simulink library "common_lib"  (R2023a)
settings: Solver=ode45  StartTime=0.0  StopTime=10.0  RelTol=1e-3
undefined symbols (not defined in the file): ACCEL_PRE_MULT, APDT_SrvcMgr_IRVHVDCSubFcnReq, C_C1GearNumbers, C_C1GearRatios, C_Calibration, C_DitherWaveform, C_GearOffset, C_GearRatioIn, C_GearRatioInverseOut, C_GearRatioOut, CLUTCH_INNER_LOOP_UPDATE_RATE, CONSTANT, DEGRADED_MODE_SIZE, Dem_EventStatusType, DiscIntNeverNeededParam, F_FAULT_ENUM, F_NOFAULT, F_OUTOFRANGE, F_RATELIMIT, FALSE, FMI14_SPECIAL_INSTRUCTIONS, FMI20_DATA_DRIFTED_HIGH, FMI21_DATA_DRIFTED_LOW, FMI29_RESERVED_FOR_SAE_ASSIGNMENT, FMI30_RESERVED_FOR_SAE_ASSIGNMENT, FMI31_CONDITION_EXISTS, FMI32_NO_FAULT, IC, k_accel, k_mean, MAX_UINT32, MEAN_PRE_MULT, NTriggers, QLTY_SIGNAL_FAILED, QLTY_SIGNAL_FULLY_FUNCTION, QLTY_SIGNAL_SUBSTITUTED_BY_1ST_CHOICE, QLTY_SIGNAL_SUBSTITUTED_BY_2ND_CHOICE, QLTY_SIGNAL_SUBSTITUTED_BY_3RD_CHOICE, QLTY_SIGNAL_SUBSTITUTED_BY_4TH_CHOICE, SAMPLE_TIME_100us, SAMPLETIME_10ms_Int, SATURATION_U16, simin, T_TestPoint, TF_FALSE, TF_TRUE, TimeStep, TRUE, WORKSPACE_UPDATE_RATE, ZERO, Zero
libraries: $bdroot x123, simulink x28, simulink_extras x4, MBD_EPS_Local_Blockset x4
(part 3 of 10)

== system common_lib/Misc ==
  note: Miscellaneous Computations
  ArcSine : Subsystem  mask(CL Trigonometric Function ArcSine){}
      mask help:
      | Simple trigonometric arcsine function.  The sine is the input and the angle is the output.
      |
      | This block is single precision.  The calculation used to determine arcsine is dervied from a Taylor Series approximation.  Note there are limitations with this approximation such as round off error.
      |
      | NgEK, Inc.
      mask Help: web(which(['common_lib51.html']))
      mask Display:
      | patch([0.30 0.30 0.70 0.70], [0.25 0.75 0.75 0.25], [255/255 127/255 255/255])
      | plot(linspace(-1,1,20)/6+0.5,(asin(linspace(-1,1,20)))/6.28+0.5)
  ClampAboveZero : Subsystem  mask(CL Clamp Above Zero){Tol=[]}
      mask prompts: Tol "Tolerance"
      mask help:
      | Clamps input above zero according to a calibratible tolerance.
      |
      | X(1) = input
      |
      | Y(1) = output
      | NgEK, Inc.
      settings: AttributesFormatString=tol=%<Tol>
      mask Help: web(which(['common_lib21.html']))
      mask Display:
      | patch([0.3 0.3 0.7 0.7], [0.35 0.65 0.65 0.35], [255/255 127/255 255/255])
      | 
      | plot([0 1],[0.5 0.5], [0.5 0.5],[0 1], [0 0.5 1], [0.55 0.55 1])
  ClampAroundZero : Subsystem  mask(CL Clamp Around Zero){Tol=[]}
      mask prompts: Tol "Tolerance"
      mask help:
      | Clamps input around zero according to a calibratible tolerance.
      |
      | X(1) = input
      |
      | Y(1) = output
      | NgEK, Inc
      mask init:
      | switch class(Tol)
      |   case ('double')
      |       One      = double(1.0);
      |        Zero     = double(0.0);
      |        MinusOne = double(-1.0);
      |  case ('single')
      |         One      = single(1.0);
      |        Zero     = single(0.0);
      |          MinusOne = single(-1.0);
      |  case ('int8')
      |         One      = int8(1.0);
      |          Zero     = int8(0.0);
      |          MinusOne = int8(-1.0);
      |     case ('int16')
      |        One      = int16(1.0);
      |         Zero     = int16(0.0);
      |         MinusOne = int16(-1.0);
      |   case ('int32')
      |         One      = int32(1.0);
      |         Zero     = int32(0.0);
      |         MinusOne = int32(-1.0);
      | end;
      settings: AttributesFormatString=tol=%<Tol>
      mask Help: web(which(['common_lib22.html']))
      mask Display:
      | patch([0.3 0.3 0.7 0.7], [0.35 0.65 0.65 0.35], [255/255 127/255 255/255])
      | 
      | plot([0 1],[0.5 0.5], [0.5 0.5],[0 1], [0 0.3 0.5 0.5 0.7 1], [0 0.3 0.3 0.7 0.7 1])
  Cosine : Subsystem  mask(CL Trigonometric Function Cosine){}
      mask help:
      | Simple trigonometric cosine function.  The angle is the input and the cosine angle is the output.
      |
      | This block is single precision.  The calculation used to determine cosine is dervied from a Taylor Series approximation.  Note there are limitations with this approximation such as round off error.
      |
      | NgEK, Inc.
      mask Help: web(which(['common_lib52.html']))
      mask Display:
      | patch([0.30 0.30 0.70 0.70], [0.25 0.75 0.75 0.25], [255/255 127/255 255/255])
      | plot(linspace(0,6.28,20)/16+0.3,(1+cos(linspace(0,6.28,20)))/4+0.25)
  Count Edges : Subsystem  mask(CL Count Edges){}
      mask help:
      | Generic counter
      |
      | Counts the number of edges from FALSE to TRUE.  Includes reset input to set the count back to zero.
      mask Help: web(which(['common_lib54.html']))
      mask Display:
      | patch([0.30 0.30 0.70 0.70], [0.25 0.75 0.75 0.25], [255/255 127/255 255/255])
      | disp('Count Edges')
  Count to X : Subsystem  mask(CL Count To X){X=[], edge=FALSE to TRUE}
      mask prompts: X "Divide by count"; edge "Count edge"
      mask help:
      | Generic count to X
      | Outputs a TRUE after X edges.
      |
      | Edge polarity and X are set by mask.
      | NgEK, Inc.
      mask init:
      | h_input      = [gcb '/Input'];
      | h_dinput    = [gcb '/DelayedInput'];
      | 
      | switch get_param(gcb,'edge')
      |    case 'FALSE to TRUE'
      |       set_param(h_input,  'Operator','AND');
      |         set_param(h_dinput, 'Operator','NAND');
      |  otherwise
      |      set_param(h_input,  'Operator','NAND');
      |         set_param(h_dinput, 'Operator','AND');
      | end
      mask Help: web(which(['common_lib26.html']))
      mask TypeOptions edge: FALSE to TRUE | TRUE to FALSE
      mask Display:
      | patch([0.1 0.1 0.9 0.9], [0.2 0.8 0.8 0.2], [255/255 127/255 255/255])
      | disp([...
      |        'Count to ' get_param(gcb,'X') '\n'...
      |        get_param(gcb,'edge')...
      |   ])
      | port_label('input',1,'in');
      | port_label('input',2,'reset?');
      | port_label('output',1,'out');
  Counter : Subsystem  mask(CL Counter){IC=[]}
      mask prompts: IC "Initial condition"
      mask help:
      | Generic counter block.
      | Counts up by up_val when count_up? is true
      | Counts down by down_val when count_down? is true.
      | Block can be used as a timer if increment value is set to the frame rate.
      |
      | X(1) = increment value
      | X(2) = count up flag
      | X(3) = decrement value
      | X(4) = count down flag
      | X(5) = max counter value
      | X(6) = min counter value
      | X(7) = reset
      |
      | Y(1) = output
      |
      | Initial condition is entered via mask.
      | NgEK, Inc.
      mask init:
      | switch class(IC)
      |    case ('double')
      |         Zero     = double(0.0);
      |   case ('single')
      |        Zero     = single(0.0);
      |   case ('int8')
      |       Zero     = int8(0.0);
      |     case ('uint16')
      |        Zero     = uint16(0.0);
      |  case ('uint32')
      |         Zero     = uint32(0.0);
      |     case ('int16')
      |         Zero     = int16(0.0);
      |    case ('int32')
      |         Zero     = int32(0.0);
      | end;
      mask Help: web(which(['common_lib23.html']))
      mask Display:
      | patch([0.4 0.4 0.6 0.6], [0.4 0.6 0.6 0.4], [255/255 127/255 255/255])
      | disp('Counter')
      | port_label('input', 1, 'up_val')
      | port_label('input', 2, 'count_up?')
      | port_label('input', 3, 'down_val')
      | port_label('input', 4, 'count_down?')
      | port_label('input', 5, 'max_count')
      | port_label('input', 6, 'min_count')
      | port_label('input', 7, 'reset?')
      | port_label('output', 1, 'output')
  Divide by X : Subsystem  mask(CL Divide By X){X=[]}
      mask prompts: X "Divide by count"
      mask help:
      | Generic divide by X
      | Outputs a true every X iterations.
      |
      | trigger? input forces output true
      |
      | Divide by X  is entered via mask.
      | NgEK, Inc.
      mask Help: web(which(['common_lib25.html']))
      mask Display:
      | patch([0.3 0.3 0.7 0.7], [0.4 0.6 0.6 0.4], [255/255 127/255 255/255])
      | disp(['Divide by ' num2str(X)])
      | port_label('input', 1, 'trigger?')
      | port_label('output', 1, 'output')
  EatonLogo : Subsystem
      mask Display: image(imread('EatonLogo.jpg'));
  EdgeTriggered Pulse : Subsystem  RTWFcnName=ETP  mask(CL Edge Triggered Pulse){Edge=TRUE to FALSE, Width=[], Pulse=TRUE, TimeStep=[], Init=0}
      mask prompts: Edge "Edge Detection"; Width "Pulse Width (seconds)"; Pulse "Pulse Value (boolean)"; TimeStep "Time Step"; Init "N/A"
      mask help:
      | Upon detection of an edge on the input (TRUE to FALSE or FALSE to TRUE)
      | output a pulse (TRUE or FALSE).
      |
      | Edge detect, pulse value, pulse width and update rate (the last two are SINGLE type) are entered via the mask.
      | NgEK, Inc.
      mask init:
      | set_param([gcb '/ETP'],'Edge',get_param(gcb,'Edge'));
      | set_param([gcb '/ETP'],'Pulse',get_param(gcb,'Pulse'));
      | set_param([gcb '/ETP'],'TimeStep',get_param(gcb,'TimeStep'));
      settings: RTWFcnNameOpts=User specified  RTWFileNameOpts=Use function name
      mask Help: web(which(['common_lib28.html']))
      mask TypeOptions Edge: FALSE to TRUE | TRUE to FALSE
      mask TypeOptions Pulse: TRUE | FALSE
      mask Display:
      | patch([0.02 0.02 0.98 0.98], [0.1 0.9 0.9 0.1], [255/255 127/255 255/255]);
      | disp([...
      |       'Edge= ' get_param(gcb,'edge') '\n'...
      |       'Width= ' get_param(gcb,'width') '\n'...
      |       'Pulse Value= ' get_param(gcb,'pulse')...
      |  ]);
  EdgeTriggered Pulse w time : Subsystem  RTWFcnName=ETPWT  mask(CL Edge Triggered Pulse w Time){Edge=TRUE to FALSE, Pulse=FALSE, TimeStep=[], Init=0}
      mask prompts: Edge "Edge Detection"; Pulse "Pulse Value (boolean)"; TimeStep "Time Step"; Init "N/A"
      mask help:
      | Upon detection of an edge on the input (TRUE to FALSE or FALSE to TRUE)
      | output a pulse (TRUE or FALSE).
      |
      | Edge detect, pulse value, pulse width and update rate (the last two are SINGLE type)
      | are entered via the mask.
      | NgEK, Inc.
      mask init:
      | switch get_param(gcb,'Edge')
      |     case 'FALSE to TRUE'
      |        TRIGGER=false;
      |    otherwise
      |        TRIGGER=true;
      | end
      | 
      | switch get_param(gcb,'Pulse')
      |    case 'FALSE'
      |       OUTPUT = false;
      |    otherwise
      |       OUTPUT = true;
      | end
      | Ts = single(TimeStep);
      | Ts_half = Ts/single(2.0);
      settings: RTWSystemCode=Inline  RTWFcnNameOpts=User specified  RTWFileNameOpts=Use function name
      mask Help: web(which(['common_lib29.html']))
      mask TypeOptions Edge: FALSE to TRUE | TRUE to FALSE
      mask TypeOptions Pulse: TRUE | FALSE
      mask Display:
      | patch([0.02 0.02 0.98 0.98], [0.1 0.9 0.9 0.1], [255/255 127/255 255/255]);
      | disp([...
      |       'Edge= ' get_param(gcb,'edge') '\n'...
      |       'Pulse Value= ' get_param(gcb,'pulse')...
      |     ]);
  GreenLeaf_Globe : Subsystem
      mask Display: image(imread('greenleaf_globe.png'));
  Hold : Subsystem  TreatAsAtomicUnit=on
      settings: RTWSystemCode=Inline
      mask Display:
      | patch([0.25 0.25 0.75 0.75], [0.05 0.3 0.3 0.05], [255/255 127/255 255/255])
      | disp('\n\nHold');
  Latch : Subsystem  mask(CL Latch){IC=[]}
      mask prompts: IC "Initial Condition"
      mask help:
      | Input is latched until reset is true
      |
      | X(1) = input
      | X(2) = reset
      |
      | Y(1) = output
      |
      | Initial condition is entered via mask.
      | NgEK, Inc.
      mask Help: web(which(['common_lib24.html']))
      mask Display:
      | patch([0.35 0.35 0.65 0.65], [0.3 0.65 0.65 0.3], [255/255 127/255 255/255])
      | disp('Latch')
      | port_label('input', 1, 'input')
      | port_label('input', 2, 'reset?')
      | port_label('output', 1, 'output')
  ModelVersion : Subsystem  mask{Parameter1=0}
      mask init:
      | % Use the simulink model verison
      | mdlName = get_param(bdroot,'name'); 
      | mdlVersionStr = get_param(bdroot,'Modelversion');
      | mdlVersion = single(str2num(mdlVersionStr));
      | mdlVersionSignal =[strrep(mdlName,'SWC_','') '_SwcVer'];
      | 
      | %Set the signal name to match the SwC
      | p = get_param([gcb '/mdlVersionBlock'],'PortHandles');
      | l = get_param(p.Outport,'Line');
      | set_param(l,'Name',mdlVersionSignal);
      | set_param(p.Outport,'MustResolveToSignalObject','on');
      | 
      | %Open the data dictionary
      | try
      |     myDictionaryObj = ...
      |     Simulink.data.dictionary.open([mdlName '.sldd']);
      |     dDataSectObj = getSection(myDictionaryObj,'Design Data');
      | 
      |     %Check if the signal object is present
      |     %foundEntries = find(dDataSectObj,'Name',mdlVersionSignal,'-class','Simulink.Signal');
      | 
      |     if ~exist(dDataSectObj,mdlVersionSignal)
      |         entryDiction = addEntry(dDataSectObj,mdlVersionSignal,Simulink.Signal);
      |         entrySub = Simulink.Signal;
      |         entrySub.DataType = 'single';
      |         entrySub.Min = 0;
      |         entrySub.CoderInfo.StorageClass = 'ExportedGlobal'
      |         setValue(entryDiction,entrySub);
      |         saveChanges(myDictionaryObj);
      |     end        
      |     close(myDictionaryObj); 
      |     
      | catch
      |     
      | end
      mask DialogControl DescTextVar Prompt: This model adds correct signal object to display the correct model version
      mask Display: disp('Model Version')
  NonZero : Subsystem  mask(CL Non Zero){Tol=0}
      mask prompts: Tol "Tolerance"
      mask help:
      | Determines whether the input is within tolerance of zero.
      |
      | Outputs a Boolean
      | TRUE means the value is non-zero
      | FALSE means the value is within tolerance of zero
      mask Display:
      | patch([0.1 0.3 0.2 0.2], [0.4 0.6 0.6 0.4], [255/255 127/255 255/255])
      | 
      | disp([...
      |       'Non-Zero\n'...
      |       'tol= ' get_param(gcb,'Tol')...
      |  ]);
  Sine : Subsystem  mask(CL Trigonometric Function Sine){}
      mask help:
      | Simple trigonometric sine function.  The angle is the input and the sine angle is the output.
      |
      | This block is single precision.  The calculation used to determine sine is dervied from a Taylor Series approximation.  Note there are limitations with this approximation such as round off error.
      |
      | NgEK, Inc.
      mask Help: web(which(['common_lib51.html']))
      mask Display:
      | patch([0.30 0.30 0.70 0.70], [0.25 0.75 0.75 0.25], [255/255 127/255 255/255])
      | plot(linspace(0,6.28,20)/16+0.3,(1+sin(linspace(0,6.28,20)))/4+0.25)
  Tangent : Subsystem  mask(CL Trigonometric Function Sine){}
      mask help:
      | Simple trigonometric tangent function.  The angle is the input and the tan angle is the output.
      |
      | This block is single precision.  The calculation used to determine tangent is dervied from a Taylor Series approximation.  Note there are limitations with this approximation such as round off error.
      |
      | NgEK, Inc.
      mask Help: web(which(['common_lib53.html']))
      mask Display:
      | patch([0.30 0.30 0.70 0.70], [0.25 0.75 0.75 0.25], [255/255 127/255 255/255])
      | plot(linspace(0,6.28,20)/16+0.3,(1+tan(linspace(0,6.28,20)))/10+0.25)
  Timeout Detection : Subsystem  RTWFcnName=TIMEOUT  mask(CL Timeout){Timeout=[], TimeStep=[]}
      mask prompts: Timeout "Timeout  (seconds)"; TimeStep "Time Step"
      mask help:
      | Timeout detection monitors the input
      | and signals a TRUE if the input is unchanging
      | for longer than the timeout interval.
      |
      | Update Rate and Timeout are entered via the mask.
      | NgEK, Inc.
      mask init:
      | % switch class(Timeout)
      | %   case ('double')
      | %        Tol      = double(TimeStep)/2.0;
      | %       Zero     = double(0.0);
      | %   case ('single')
      | %         Tol      = single(double(TimeStep)/2.0);
      | %         Zero     = single(0.0);
      | %    case ('int8')
      | %       Tol      = int8(double(TimeStep)/2.0);
      | %          Zero     = int8(0.0);
      | %     case ('int16')
      | %         Tol      = int16(double(TimeStep)/2.0);        
      | %       Zero     = int16(0.0);
      | %    case ('int32')
      | %          Tol      = int32(double(TimeStep)/2.0);       
      | %        Zero     = int32(0.0);
      | % end;
      | 
      | Ts = single(TimeStep);
      | Tol = Ts/single(2.0);
      | Zero = single(0.0);
      settings: RTWFcnNameOpts=User specified  RTWFileNameOpts=Use function name
      mask Help: web(which(['common_lib27.html']))
      mask Display:
      | patch([0.05 0.05 0.95 0.95], [0.15 0.85 0.85 0.15], [255/255 127/255 255/255]);
      | disp(['Timeout = \n' get_param(gcb,'Timeout')]);
  Timeout with time : Subsystem  RTWFcnName=TIMEOUT  mask(CL Timeout){TimeStep=[]}
      mask prompts: TimeStep "Time Step"
      mask help:
      | Timeout detection monitors the input
      | and signals a TRUE if the input is unchanging
      | for longer than the timeout interval.
      |
      | Update Rate and Timeout are entered via the mask.
      | NgEK, Inc.
      mask init: same as common_lib/Misc/Timeout Detection
      settings: RTWFcnNameOpts=User specified  RTWFileNameOpts=Use function name
      mask Help: web(which(['common_lib27.html']))
      mask Display:
      | patch([0.05 0.05 0.95 0.95], [0.15 0.85 0.85 0.15], [255/255 127/255 255/255]);
      | disp(['Timeout = \n Input Port 2' ]);
  Timeout with time Integer : Subsystem  RTWFcnName=TIMEOUT  mask(CL Timeout){TimeStep=[]}
      mask prompts: TimeStep "Time Step"
      mask help:
      | Timeout detection monitors the input
      | and signals a TRUE if the input is unchanging
      | for longer than the timeout interval.
      |
      | Update Rate and Timeout are entered via the mask.
      | NgEK, Inc.
      mask init:
      | % switch class(Timeout)
      | %   case ('double')
      | %        Tol      = double(TimeStep)/2.0;
      | %       Zero     = double(0.0);
      | %   case ('single')
      | %         Tol      = single(double(TimeStep)/2.0);
      | %         Zero     = single(0.0);
      | %    case ('int8')
      | %       Tol      = int8(double(TimeStep)/2.0);
      | %          Zero     = int8(0.0);
      | %     case ('int16')
      | %         Tol      = int16(double(TimeStep)/2.0);        
      | %       Zero     = int16(0.0);
      | %    case ('int32')
      | %          Tol      = int32(double(TimeStep)/2.0);       
      | %        Zero     = int32(0.0);
      | % end;
      | 
      | Ts = uint16(TimeStep);
      | Tol = uint16(Ts/uint16(2));
      | Zero = uint16(0);
      settings: RTWFcnNameOpts=User specified  RTWFileNameOpts=Use function name
      mask Help: web(which(['common_lib27.html']))
      mask Display:
      | patch([0.05 0.05 0.95 0.95], [0.15 0.85 0.85 0.15], [255/255 127/255 255/255]);
      | disp(['Int_Timeout = \n Input Port 2' ]);
  Value Latch1 : Subsystem  mask(CL Latch){IC=[], HoldTime=0, TimeStep=0}
      mask prompts: IC "Initial Condition"; HoldTime "Hold Time"; TimeStep "Time Step"
      mask help:
      | Input is latched until reset is true
      |
      | X(1) = input
      | X(2) = reset
      |
      | Y(1) = output
      |
      | Initial condition is entered via mask.
      | NgEK, Inc.
      mask Help: web(which(['common_lib24.html']))
      mask Display:
      | patch([0.35 0.35 0.65 0.65], [0.3 0.65 0.65 0.3], [255/255 127/255 255/255])
      | disp('Latch')
      | port_label('input', 1, 'input')
      | port_label('output', 1, 'output')

== system common_lib/OS ==
  note: These components are atomic elements used by the
      | schedule_morph script to build scheduler blocks
  note: OS Components
  Scheduler : Subsystem  mask(CL Scheduler){Number=5, DType=Fcn_Call, Style=Trigger all tasks each frame, State=off}
      mask prompts: Number "Number of Tasks to Trigger"; DType "Type of Trigger"; Style "Schedule Style"; State "Display Scheduler State"
      mask help:
      | Simulink-based task scheduler capable of generating  boolean or fcn_call triggers.  Tasks may be staggered so that one is executed each frame in a round-robin fashion or all tasks may be triggered in sequence in a single frame.
      |
      | Boolean output for all tasks triggering in a frame is not implemented yet.
      |
      | NgEK, Inc.
      mask init:
      | NTriggers=int8(max([Number 1]));
      | TRUE = boolean(1);
      | FALSE = boolean(0);
      | schedule_morph;
      settings: RTWSystemCode=Nonreusable function  RTWFcnNameOpts=Use subsystem name  RTWFileNameOpts=Use subsystem name
      mask Help: web(which(['common_lib30.html']))
      mask TypeOptions DType: Boolean | Fcn_Call
      mask TypeOptions Style: Trigger one task per frame | Trigger all tasks each frame
      mask Display:
      | patch([0.3 0.3 0.7 0.7], [0.35 0.65 0.65 0.35], [255/255 127/255 255/255])
      | disp('Scheduler');
      | 
      | port_label('output',1,'Task 1');
      | port_label('output',2,'Task 2');
      | port_label('output',3,'Task 3');
      | port_label('output',4,'Task 4');
      | port_label('output',5,'Task 5');
  Scheduler with Init : Subsystem  mask(CL Scheduler with Init){Number=2}
      mask prompts: Number "Number of Tasks to Trigger"
      mask help:
      | Simulink-based task scheduler capable of generating  fcn_call triggers.  Tasks are triggered in sequence in a single frame.  The task wired to the "Init" port is only executed in the first frame.
      |
      | NgEK, Inc.
      mask init:
      | NTriggers=int8(max([Number 1]));
      | TRUE = boolean(1);
      | FALSE = boolean(0);
      | schedule_morph2;
      settings: RTWSystemCode=Nonreusable function  RTWFcnNameOpts=Use subsystem name  RTWFileNameOpts=Use subsystem name
      mask Help: web(which(['common_lib55.html']))
      mask Display:
      | patch([0.3 0.3 0.7 0.7], [0.35 0.65 0.65 0.35], [255/255 127/255 255/255])
      | disp('Scheduler\nwith Init');
      | 
      | port_label('output',1,'Init');
      | port_label('output',2,'Task 1');
      | port_label('output',3,'Task 2');
  fcn_call generator : Subsystem  TreatAsAtomicUnit=on
  schedule counter : Subsystem
  sequence generator : Subsystem  TreatAsAtomicUnit=on

== system common_lib/SCond ==
  note: Signal Conditioning
  Gain and Offset (in) : Subsystem  mask(CL Gain And Offset (in)){DataType=Single}
      mask prompts: DataType "Output Data Type"
      mask help:
      | Gain/Offset with data type coercion
      |
      | NgEK, Inc.
      mask init:
      | h=gcb;
      | 
      | set_param([h '/InputConversion'], 'DataType','single');
      | set_param([h '/InputConversion1'], 'DataType','single');
      | set_param([h '/InputConversion2'], 'DataType','single');
      | 
      | switch DataType
      |   case (1)
      |       set_param([h '/OutputConversion'], 'DataType','int8');
      |  case (2)
      |       set_param([h '/OutputConversion'], 'DataType','uint8');
      |    case (3)
      |       set_param([h '/OutputConversion'], 'DataType','int16');
      |  case (4)
      |      set_param([h '/OutputConversion'], 'DataType','uint16');
      |   case (5)
      |         set_param([h '/OutputConversion'], 'DataType','single');
      |    case (6)
      |         set_param([h '/InputConversion'], 'DataType','double');
      |         set_param([h '/InputConversion1'], 'DataType','double');
      |         set_param([h '/InputConversion2'], 'DataType','double');
      |      set_param([h '/OutputConversion'], 'DataType','double');    
      |    otherwise
      |      set_param([h '/OutputConversion'], 'DataType','single');
      | end
      mask Help: web(which(['common_lib32.html']))
      mask TypeOptions DataType: Int8 | UInt8 | Int16 | UInt16 | Single | Double
      mask Display:
      | patch([0.35 0.35 0.65 0.65], [0.35 0.65 0.65 0.35], [255/255 127/255 255/255]);
      | disp(['mx-b']);
  Gain and Offset (out) : Subsystem  mask(CL Gain And Offset (out)){DataType=Single}
      mask prompts: DataType "Output Data Type"
      mask help:
      | Gain/Offset with data type coercion
      |
      | NgEK, Inc.
      mask init: same as common_lib/SCond/Gain and Offset (in)
      mask Help: web(which(['common_lib33.html']))
      mask TypeOptions DataType: Int8 | UInt8 | Int16 | UInt16 | Single | Double
      mask Display:
      | patch([0.35 0.35 0.65 0.65], [0.35 0.65 0.65 0.35], [255/255 127/255 255/255]);
      | disp(['(x+b)/m']);
  Membership Function : Subsystem  mask(CL Membership Function){Low=single(10), Peak=single(50), High=single(90), DType=Upper Trapezoid}
      mask prompts: Low "Lower Value"; Peak "Peak Value"; High "Upper Value"; DType "Membership Type"
      mask help:
      | Triangular membership function calculation with an output of 1 at the "Peak" value and dropping off to 0 towards the "Low" and "High" values.  End "trapezoid" membership functions may be specified with the membership "type" pulldown menu.
      |
      | X(1) = Independent Variable
      |
      | Y(1) = Membership Function (0:1)
      |
      | NgEK, Inc.
      mask init:
      | if Peak<Low | Peak>High, disp(['WARNING: Breakpoints Non-Monotonic in <' gcb '>!']), end
      | 
      | switch class(Peak)
      |   case ('double')
      |        Zero      = double( 0.0);
      |          One       = double( 1.0);
      |         if (DType==1)
      |             SlopeLow  = 0.0;
      |           SlopeHigh = 1.0/(Peak-High);
      |         elseif (DType==2)
      |             SlopeLow  = 1.0/(Peak-Low);
      |            SlopeHigh = 1.0/(Peak-High);
      |       else
      |          SlopeLow  = 1.0/(Peak-Low);
      |           SlopeHigh = 0.0;
      |        end;
      |      
      |     case ('single')
      |        Zero      = single( 0.0);
      |          One       = single( 1.0);
      |        if (DType==1)
      |            SlopeLow  = single(0.0);
      |           SlopeHigh = single(1.0/(double(Peak)-double(High)));
      |          elseif (DType==2)
      |            SlopeLow  = single(1.0/(double(Peak)-double(Low)));
      |            SlopeHigh = single(1.0/(double(Peak)-double(High)));
      |       else
      |          SlopeLow  = single(1.0/(double(Peak)-double(Low)));
      |           SlopeHigh = single(0.0);
      |         end;
      | end;
      | 
      | if     (abs(double(SlopeLow))<abs(double(SlopeHigh)))
      |   XPltAxis = [ 0 0.2 0.7 0.8 1.0 ];
      | elseif (abs(double(SlopeHigh))<abs(double(SlopeLow)))
      |  XPltAxis = [ 0 0.2 0.3 0.8 1.0 ];
      | else
      |  XPltAxis = [ 0 0.2 0.5 0.8 1.0 ];
      | end;
      | 
      | if     (DType==1)
      |        YPltAxis = [ 1 1 0 0 0 ];
      | elseif (DType==2)
      |        YPltAxis = [ 0 0 1 0 0 ];
      | else
      |        YPltAxis = [ 0 0 0 1 1 ];
      | end;
      mask Help: web(which(['common_lib36.html']))
      mask TypeOptions DType: Lower Trapezoid | Central Triangle | Upper Trapezoid
      mask Display:
      | patch([.2 .2 .8 .8],[.2 .85 .85 .2],[255/255 127/255 255/255])
      | plot(XPltAxis, YPltAxis);
      | disp(['Low=',num2str(double(Low)),sprintf('\n'),'Peak=',num2str(double(Peak)),sprintf('\n'),'High=',num2str(double(High))])
  Test Override Gain and Offset (in) : Subsystem  mask(CL Gain And Offset (in)){DataType=Single}
      mask prompts: DataType "Output Data Type"
      mask help: Gain/Offset with enabled Gain and Offset option and with Output data type conversion
      mask init: same as common_lib/SCond/Gain and Offset (in)
      mask TypeOptions DataType: Int8 | UInt8 | Int16 | UInt16 | Single | Double
      mask Display:
      | patch([0.3 0.3 0.7 0.7], [0.35 0.65 0.65 0.35], [255/255 127/255 255/255])
      | disp(['Y=mX+b\nTest Override'])
  ramp to zero : Subsystem  mask(CL Ramp to Zero){DataType=Single}
      mask prompts: DataType "Data Type"
      mask help:
      | Ramp input signal to zero
      |
      | X(1) = Speed
      | X(2) = Limit
      |
      | Y(1) = Factor
      |
      | NgEK, Inc.
      mask init:
      | switch DataType
      |     case (1)
      |        One      = single( 1.0);
      |          MinusOne = single(-1.0);
      |         Zero     = single( 0.0);
      |     case (2)
      |         One      = double( 1.0);
      |          MinusOne = double(-1.0);
      |       Zero     = double( 0.0);
      | end;
      mask Help: web(which(['common_lib34.html']))
      mask TypeOptions DataType: Single | Double
      mask Display:
      | patch([0.3 0.3 0.7 0.7], [0.3 0.7 0.7 0.3], [255/255 127/255 255/255]);
      | disp('ramp to\nzero')

== system common_lib/Signal Conditioning ==
  note: Signal Conditioning
  2nd Order Butterworth Filter : Subsystem  mask{IC=0, TSAMP=0}
      mask prompts: IC "Initial Condition"; TSAMP "Sample Time"
      mask Display:
      | patch([0.35 0.35 0.65 0.65], [0.3 0.7 0.7 0.3], [255/255 127/255 255/255])
      | disp('2nd Order\nButterworth')
      | port_label('input',1,'input')
      | port_label('input',2,'cutoff_freq')
      | port_label('input',3,'reset')
      | port_label('output',1,'output')
  AnalogChecking : Subsystem  TreatAsAtomicUnit=on  mask{TimeStep=[]}
      mask prompts: TimeStep "Time Step"
  DitherSaturation : Subsystem  Description=|
      | This block generates dither using the table given for DitherWaveform at the frequency and amplitude given by the freq_hz and amplitude inputs.  All inputs should be 'single' datatype.  The table should be 'single' data type also.  The block runs at the sample time of the 'in' input.  It generates the correct frequency dither regardless of sample time.
      |                                                                                                                                                                                                                                                                                                                                                                  
      | Since it may not be possible to generate the exact frequency specified in the 'freq_hz' input, the block puts out the actual frequency in the 'realized_frequency' output.
  DitherSaturation1 : Subsystem  Description=|
      | This block generates dither using the table given for DitherWaveform at the frequency and amplitude given by the freq_hz and amplitude inputs.  All inputs should be 'single' datatype.  The table should be 'single' data type also.  The block runs at the sample time of the 'in' input.  It generates the correct frequency dither regardless of sample time.
      |                                                                                                                                                                                                                                                                                                                                                                  
      | Since it may not be possible to generate the exact frequency specified in the 'freq_hz' input, the block puts out the actual frequency in the 'realized_frequency' output.
  HydValveDither : Subsystem  Description=|  mask{DitherWaveform=single(C_DitherWaveform), ts=0}
      | This block generates dither using the table given for DitherWaveform at the frequency and amplitude given by the freq_hz and amplitude inputs.  All inputs should be 'single' datatype.  The table should be 'single' data type also.  The block runs at the sample time of the 'in' input.  It generates the correct frequency dither regardless of sample time.
      |                                                                                                                                                                                                                                                                                                                                                                  
      | Since it may not be possible to generate the exact frequency specified in the 'freq_hz' input, the block puts out the actual frequency in the 'realized_frequency' output.
      mask prompts: DitherWaveform "Dither Waveform"; ts "Sample Time"
  Normalized Variable Tanh Curve : Subsystem  mask{TimeStep=TimeStep}
      mask prompts: TimeStep "Sample Time"
      mask Display:
      | patch([0.3 0.3 0.7 0.7], [0.35 0.65 0.65 0.35], [255/255 127/255 255/255])
      | plot([0:.05:1],(tanh(([0:.05:1]*2*pi)-pi)+1)/2)
      | port_label('input',1,'RampTime')
      | port_label('input',2,'Reset')
      | port_label('output',1,'Out')
  Obsolete Signal Conditioning : Subsystem
      mask Display: disp('Obsolete\nSignal\nConditioning')
  OffsetAndGain : Subsystem  TreatAsAtomicUnit=on  mask(CL_OffsetAndGain){}
      mask help: Gain/Offset
      mask Help: web(which(['common_lib32.html']))
      mask Display:
      | patch([0.3 0.3 0.7 0.7], [0.4 0.6 0.6 0.4], [205/255 205/255 255/255]);
      | disp(['m*(x+b)']);
  SpeedProcess : Subsystem
  Trajectory : Subsystem  mask{TimeStep=TimeStep, wn=single(30), damping=single(.8)}
      mask prompts: TimeStep "Sample Time"; wn "Natural Frequency"
      mask Display:
      | patch([0.325 0.325 0.675 0.675], [0.35 0.65 0.65 0.35], [255/255 127/255 255/255])
      | disp('Trajectory')
      | port_label('input',1,'In')
      | port_label('input',2,'MaxAccel')
      | port_label('input',3,'MinAccel')
      | port_label('input',4,'MaxJerk')
      | port_label('input',5,'MinJerk')
      | port_label('input',6,'Reset')
      | port_label('output',1,'Out')
  Variable Tanh Curve : Subsystem  mask{TimeStep=TimeStep}
      mask prompts: TimeStep "Sample Time"
      mask Display:
      | patch([0.3 0.3 0.7 0.7], [0.35 0.65 0.65 0.35], [255/255 127/255 255/255])
      | plot([0:.05:1],(tanh(([0:.05:1]*2*pi)-pi)+1)/2)
      | port_label('input',1,'StartValue')
      | port_label('input',2,'FinalValue')
      | port_label('input',3,'RampTime')
      | port_label('input',4,'Reset')
      | port_label('output',1,'Out')
      | port_label('output',2,'RampComplete')

== system common_lib/Signal Generators ==
  note: Signal Generators
  Clu_2_1_3_1_1_1_TestSignalBuilder : Subsystem
  CustomProfileGenerator : Subsystem  mask{TimeStep=single(0.002)}
      mask prompts: TimeStep "Time Step"
  Signal Generator Components : Subsystem
      mask Display: disp('Signal\nGenerators\nComponents')
  SquareTriangleWaveDither : Subsystem  mask{TimeStep=single(0.002)}
      mask prompts: TimeStep "Time Step"
  SquareTriangleWaveDitherPWM : Subsystem  mask{TimeStep=single(0.002)}
      mask prompts: TimeStep "Time Step"
  SquareTriangleWaveGenerator_Advanced : Subsystem  mask{TimeStep=0}
      mask prompts: TimeStep "Time Step"
  SquareTriangleWaveGenerator_Basic : Subsystem  mask{TimeStep=0}
      mask prompts: TimeStep "Time Step"

== system common_lib/Signal Routing ==
  note: Signal Routing
  Overwrite : Subsystem  mask{VarName=VariableName, OverwriteEnable=off, OverwriteValue=0}
      mask prompts: VarName "Name"; OverwriteEnable "Overwrite ?"; OverwriteValue "Value"
      mask init:
      | enabled = strncmpi(get_param(gcb, 'OverwriteEnable'), 'on', 2);
      | 
      | if (enabled)
      |     dispname = char(get_param(gcb, 'OverwriteValue'));
      | else
      |     dispname = char('No Overwrite');
      | end
      | 
      | dispname = [VarName '\n' dispname];
      | 
      | %
      | % Change the name of the constants to match the VarName
      | %
      | rtblockname = char(find_system(gcb, 'LookUnderMasks', 'all', 'FollowLinks', 'on', 'BlockType', 'Constant'));
      | 
      | % The first constant should be the overwrite enable
      | set_param(deblank(rtblockname(1,:)), 'Name', strcat('xPCOE_', VarName));
      | 
      | % The second constant should be the overwrite value
      | set_param(deblank(rtblockname(2,:)), 'Name', strcat('xPCOV_', VarName));
      mask Display: disp(dispname)
  Vector to Bus : Subsystem  mask(Vector To Bus){BOName=BO_}
      mask prompts: BOName "Bus Object Name (Must be in workspace)"
      mask help:
      | This block takes in a vector and adds the signal names specified in the bus
      | object.  The output is a bus.
      |
      | In the present state of development this block only works for 8 input elements.
      mask init:
      | % Set the number of signals in the input mux.  This should really come from
      | % the dialog box. 
      | NumInputs = 8;
      | 
      | % Get the name of the bus object
      | BOName = get_param(gcb, 'BOName');
      | 
      | % If this workspace var is not of type Simulink.Bus there is a problem
      | a = evalin('base', ['whos(''' BOName ''')']);
      | 
      | if (length(a)==0) 
      |     error('The dialog must specify a valid Simulink.Bus')
      | end
      | if (strcmp(a.class, 'Simulink.Bus')==0)
      |     error('The dialog must specify a valid Simulink.Bus')
      | end
      | 
      | % Find the number of elements in the bus object
      | BONumelm = evalin('base', ['length(' BOName '.Elements)']);
      | 
      | % Get the names from the bus object
      | for x=1:BONumelm
      |     SigNames{x} = evalin('base', [BOName '.Elements(' sprintf('%i',x) ').Name']);
      | end
      | 
      | % Find the bus creator
      | BusCreator = char(find_system(gcb, 'LookUnderMasks', 'all', 'FollowLinks', 'on', 'BlockType', 'BusCreator'));
      | p = get_param(BusCreator, 'PortHandles');
      | l = get_param(p.Inport, 'Line');
      | 
      | % Assign the names to the signals going into the bus creator
      | for x=1:NumInputs
      |     if (x<=BONumelm)
      |        set_param(l{x}, 'Name', SigNames{x});
      |     else
      |        set_param(l{x}, 'Name', sprintf('Signal%i', x));
      |     end
      | end
      mask Display: disp(BOName)

== system common_lib/Slink ==
  note: Simulink Enhancements
  Dead : Subsystem  mask(CL Variable Deadband){DataType=Single}
      mask prompts: DataType "Data Type"
      mask help:
      | Deadband with smooth output transition from deadband region.
      |
      | X(1) = input
      | X(2) = deadband
      |
      | Y(1) = output
      | NgEK, Inc.
      mask init:
      | switch DataType
      |     case (1)
      |        Zero     = double( 0.0);
      |          MinusOne = double(-1.0);
      |     case (2)
      |          Zero     = single( 0.0);
      |       MinusOne = single(-1.0);
      |    case (3)
      |        Zero     = int8( 0.0);
      |         MinusOne = int8(-1.0);
      |     case (4)
      |        Zero     = int16( 0.0);
      |       MinusOne = int16(-1.0);
      |     case (5)
      |          Zero     = int32( 0.0);
      |          MinusOne = int32(-1.0);
      | end;
      mask Help: web(which(['common_lib35.html']))
      mask TypeOptions DataType: Double | Single | Int8 | Int16 | Int32
      mask Display:
      | patch([0.3 0.3 0.7 0.7], [0.35 0.65 0.65 0.35], [255/255 127/255 255/255])
      | 
      | plot([0 1],[0.5 0.5], [0.5 0.5],[0 1], [0.1 0.35],[0.1 0.5], [0.65 0.9],[0.5 0.9])
  Hysteresis : Subsystem  mask(CL Hysteresis){IC=[]}
      mask prompts: IC "Initial Condition"
      mask help:
      | Hysteresis block
      |
      | X(1) = Input
      | X(2) = Deadband Width
      |
      | Y(1) = Output
      | NgEK, Inc.
      mask init:
      | switch class(IC)
      |    case ('double')
      |         MinusOne = double(-1.0);
      |  case ('single')
      |        MinusOne = single(-1.0);
      |  case ('int8')
      |       MinusOne = int8(-1.0);
      |     case ('int16')
      |       MinusOne = int16(-1.0);
      |     case ('int32')
      |          MinusOne = int32(-1.0);
      | end;
      mask Help: web(which(['common_lib42.html']))
      mask Display:
      | patch([0.3 0.3 0.7 0.7], [0.35 0.65 0.65 0.35], [255/255 127/255 255/255])
      | 
      | plot([0 .6 .75 1],[.25 .25 .75 .75], [.25 .4 .75],[.25 .75 .75], [.4 .5 .4],[.35 .25 .15], [.6 .5 .6],[.85 .75 .65])
  Relay : Subsystem  mask(CL Relay){init=[]}
      mask prompts: init "Initiailization State"
      mask help:
      | Relay block
      |
      | X(1) = Input
      | X(2) = Upper Threshold
      | X(3) = Lower Threshold
      | X(4) = Upper Value
      | X(5) = Lower Value
      |
      | Y(1) = output
      | NgEK, Inc.
      mask Help: web(which(['common_lib41.html']))
      mask Display:
      | patch([0.3 0.3 0.7 0.7], [0.35 0.65 0.65 0.35], [255/255 127/255 255/255])
      | 
      | plot([0 .75 .75 1],[.25 .25 .75 .75], [.25 .25 .75],[.25 .75 .75], [.4 .5 .4],[.35 .25 .15], [.6 .5 .6],[.85 .75 .65])
  Relay_1 : Subsystem  mask(CL Relay){}
      mask help:
      | Relay block
      |
      | X(1) = Input
      | X(2) = hysterisis
      | X(3) = Ending Point
      | Y(1) = output
      | NgEK, Inc.
      mask Help: web(which(['common_lib41.html']))
      mask Display:
      | patch([0.3 0.3 0.7 0.7], [0.35 0.65 0.65 0.35], [255/255 127/255 255/255])
      | 
      | plot([0 .75 .75 1],[.25 .25 .75 .75], [.25 .25 .75],[.25 .75 .75], [.4 .5 .4],[.35 .25 .15])
      | 
      | port_label('input', 1, 'Input')
      | port_label('input', 2, 'dead band')
      | port_label('input', 3, 'B')
      | port_label('output', 1, 'out')
  Sat : Subsystem  mask(CL Variable Saturation){}
      mask help:
      | Variable saturation block
      |
      | X(1) = input
      | X(2) = upper limit
      | X(3) = lower limit
      |
      | Y(1) = output
      | NgEK, Inc.
      mask Help: web(which(['common_lib37.html']))
      mask Display:
      | patch([0.3 0.3 0.7 0.7], [0.35 0.65 0.65 0.35], [255/255 127/255 255/255])
      | 
      | plot([0 1],[0.5 0.5],[0.5 0.5],[0 1],[0 0.25 0.75 1],[0 0 1 1])
  Three Value Threshold : Subsystem  mask(CL ThreeValuedThreshold){}
      mask help:
      | Relay block
      |
      | X(1) = Input
      | X(2) = Upper Threshold
      | X(3) = Lower Threshold
      | X(4) = Upper Value
      | X(5) = Between Value
      | X(6) = Lower Value
      |
      | Y(1) = output
      | NgEK, Inc.
      mask Help:
      | Relay block
      | 
      | X(1) = Input
      | X(2) = Upper Threshold
      | X(3) = Lower Threshold
      | X(4) = Upper Value
      | X(5) = Between Value
      | X(6) = Lower Value
      | 
      | Y(1) = output
      | NgEK, Inc.
      mask Display:
      | patch([0.3 0.3 0.7 0.7], [0.35 0.65 0.65 0.35], [255/255 127/255 255/255])
      | 
      | plot([0 0.25 0.25 0.75 0.75 1],[0.25 0.25 0.5 0.5 0.75 0.75]);
      | 
      | %plot([0 .75 .75 1],[.25 .25 .75 .75], [.25 .25 .75],[.25 .75 .75], [.4 .5 .4],[.35 .25 .15], [.6 .5 .6],[.85 .75 .65])
  Variable Rate Limiter : Subsystem  mask(CL Variable Rate Limiter){TimeStep=[], ic=[]}
      mask prompts: TimeStep "Time Step"; ic "Initial Condition"
      mask help:
      | Variable rate limiter block
      |
      | X(1) = input
      | X(2) = rise rate
      | X(3) = fall rate
      |
      | Y(1) = output
      | NgEK, Inc.
      mask Help: web(which(['common_lib38.html']))
      mask Display:
      | patch([0.3 0.3 0.7 0.7], [0.35 0.65 0.65 0.35], [255/255 127/255 255/255])
      | 
      | plot([0 1],[0.5 0.5],[0.5 0.5],[0 1],[0 1],[0 1],[0.7 0.8 0.8],[0.8 0.8 0.7], [0.2 0.2 0.3],[0.3 0.2 0.2])
  Variable Rate Limiter w IC : Subsystem  mask(CL Variable Rate Limiter with Initial Condition){TimeStep=[], ic=[]}
      mask prompts: TimeStep "Time Step"; ic "Initial Condition"
      mask help:
      | Variable rate limiter block with Initial Condiiton
      |
      | X(1) = input
      | X(2) = rise rate
      | X(3) = fall rate
      | X(4) = initial condition
      | X(5) = reset?
      |
      | Y(1) = output
      | NgEK, Inc.
      mask Help: web(which(['common_lib39.html']))
      mask Display:
      | patch([0.3 0.3 0.7 0.7], [0.35 0.65 0.65 0.35], [255/255 127/255 255/255])
      | 
      | plot([0 1],[0.5 0.5],[0.5 0.5],[0 1],[0 1],[0 1],[0.7 0.8 0.8],[0.8 0.8 0.7], [0.2 0.2 0.3],[0.3 0.2 0.2])
  Variable Rate Limiter w IC and Sat : Subsystem  mask(CL Variable Rate Limiter with IC and Saturation){TimeStep=[], ic=[]}
      mask prompts: TimeStep "Time Step"; ic "Initial Condition"
      mask help:
      | Variable rate limiter block with Initial Condition and Saturation
      |
      | X(1) = input
      | X(2) = rise rate
      | X(3) = fall rate
      | X(4) = upper limit
      | X(5) = lower limit
      | X(6) = initial condition
      | X(7) = reset?
      |
      | Y(1) = output
      | NgEK, Inc.
      mask Help: web(which(['common_lib40.html']))
      mask Display:
      | patch([0.3 0.3 0.7 0.7], [0.35 0.65 0.65 0.35], [255/255 127/255 255/255])
      | 
      | plot([0 1],[0.5 0.5],[0.5 0.5],[0 1],[0 0.25 0.75 1],[0 0 1 1],[0.3 0.3 0.45],[0.25 0.1 0.2],[0.55 0.7 0.75],[0.8 0.9 0.78])

== system common_lib/Tbl ==
  note: Tables
  2D Lookup : Subsystem  TreatAsAtomicUnit=on  RTWFcnName=VARTABLE  mask(CL 2D Table Lookup){}
      mask help:
      | 2D Table lookup with explicit axis inputs. Utilize  standard Simulink Prelookup table (2019a).
      |
      | X(1) = Independent variable
      | X(2) = Breakpoint
      | X(3) = Table Data
      |
      | Y(1) = output
      settings: RTWFcnNameOpts=User specified  RTWFileNameOpts=Use function name
      mask Help: web(which(['common_lib45.html']))
      mask Display:
      | patch([0.3 0.3 0.7 0.7], [0.35 0.65 0.65 0.35], [255/255 127/255 255/255])
      | 
      | plot([0.2 0.2],[0.2 0.8],[0.2 0.8],[0.2 0.2],linspace(0.2,0.8,10),0.2+0.8*linspace(0.2,0.8,10).^2)
  Direct Look-Up Table (n-D) : LookupNDDirect
      settings: AttributesFormatString=%<mxTable>
  Interpolator : Subsystem  mask(CL Interpolation){DType=Double}
      mask prompts: DType "Data Type"
      mask help:
      | 1D Interpolation Block
      |
      | X(1) = value at 1
      | X(2) = value at 0
      | X(3) = interpolation value
      |
      | Y(1) = output
      | NgEK, Inc.
      mask init:
      | switch DType
      |    case (1)
      |       set_param([gcb '/XY Interpolator'],'DType','double');
      |        Zero = double(0.0);
      |          One  = double(1.0);
      |     case (2)
      |        set_param([gcb '/XY Interpolator'],'DType','single');
      |         Zero = single(0.0);
      |        One  = single(1.0);
      | end;
      mask Help: web(which(['common_lib43.html']))
      mask TypeOptions DType: Double | Single
      mask Display:
      | patch([0.3 0.3 0.7 0.7], [0.35 0.65 0.65 0.35], [255/255 127/255 255/255])
      | 
      | plot([.2 .9],[0.5 0.5],[0.2 0.3 0.8 .9],[.25 .25 .75 .75])
      | 
      | port_label('input', 1, '1')
      | port_label('input', 2, '0')
      | port_label('input', 3, 'interp')
  Look-Up Table : Lookup  InputValues=[-5:5]  Table=tanh([-5:5])  LookUpMeth=Interpolation-Use End Values  SaturateOnIntegerOverflow=off
      settings: AttributesFormatString=%<OutputValues>
  Look-Up Table (2-D) : Lookup2D  RowIndex=[1:3]  ColumnIndex=[1:3]  Table=[4 5 6;16 19 20;10 18 23]  LookUpMeth=Interpolation-Use End Values  SaturateOnIntegerOverflow=off  InputSameDT=off
      settings: AttributesFormatString=%<OutputValues>
  XY Interpolator : Subsystem  TreatAsAtomicUnit=on  RTWFcnName=XYINT  mask(CL XY Interpolation){DType=single}
      mask prompts: DType "Data Type"
      mask help:
      | 2D Interpolation Block
      |
      | X(1) = output value at 1
      | X(2) = output value at 0
      | X(3) = input value corresponding to 1
      | X(4) = input value corresponding to 0
      | X(5) = input value
      |
      | Y(1) = output
      | NgEK, Inc.
      mask init:
      | switch DType
      |    case (1)
      |       set_param([gcb '/Interp'],...
      |          'FunctionName','xyinterp_f64_wrap',...
      |           'SFunctionModules','xyinterp_f64');
      | %        Zero = double(0.0);
      | %          One  = double(1.0);
      | %        Tol  = double(1e-6);
      |     case (2)
      |        set_param([gcb '/Interp'],...
      |           'FunctionName','xyinterp_f32_wrap',...
      |           'SFunctionModules','xyinterp_f32');
      | %        Zero = single(0.0);
      | %        One  = single(1.0);
      | %         Tol  = single(1e-6);
      | end;
      | % strDType = get_param(gcb,'DType');
      | % set_param([gcb '/DTC'],'OutDataTypeStr',strDType);
      | % set_param([gcb '/DTC1'],'OutDataTypeStr',strDType);
      | % set_param([gcb '/DTC2'],'OutDataTypeStr',strDType);
      | % set_param([gcb '/DTC3'],'OutDataTypeStr',strDType);
      | % set_param([gcb '/DTC4'],'OutDataTypeStr',strDType);
      settings: RTWFcnNameOpts=User specified  RTWFileNameOpts=Use function name
      mask Help: web(which(['common_lib44.html']))
      mask TypeOptions DType: double | single
      mask Display:
      | patch([0.3 0.3 0.7 0.7], [0.35 0.65 0.65 0.35], [255/255 127/255 255/255])
      | 
      | plot([.2 .9],[0.5 0.5],[0.2 0.3 0.8 .9],[.25 .25 .75 .75])
      | 
      | port_label('input', 1, 'Y_1')
      | port_label('input', 2, 'Y_0')
      | port_label('input', 3, 'X_1')
      | port_label('input', 4, 'X_0')
      | port_label('input', 5, 'X')
  XY Interpolator1 : Subsystem  TreatAsAtomicUnit=on  RTWFcnName=XYINT  mask(CL XY Interpolation){DType=single}
      mask prompts: DType "Data Type"
      mask help:
      | 2D Interpolation Block
      |
      | X(1) = output value at 1
      | X(2) = output value at 0
      | X(3) = input value corresponding to 1
      | X(4) = input value corresponding to 0
      | X(5) = input value
      |
      | Y(1) = output
      | NgEK, Inc.
      mask init:
      | switch DType
      |    case (1)
      |        Zero = double(0.0);
      |          One  = double(1.0);
      |        Tol  = double(1e-6);
      |     case (2)
      |        Zero = single(0.0);
      |        One  = single(1.0);
      |         Tol  = single(1e-6);
      | end;
      | strDType = get_param(gcb,'DType');
      | set_param([gcb '/DTC'],'OutDataTypeStr',strDType);
      | set_param([gcb '/DTC1'],'OutDataTypeStr',strDType);
      | set_param([gcb '/DTC2'],'OutDataTypeStr',strDType);
      | set_param([gcb '/DTC3'],'OutDataTypeStr',strDType);
      | set_param([gcb '/DTC4'],'OutDataTypeStr',strDType);
      settings: RTWSystemCode=Inline  RTWFcnNameOpts=User specified  RTWFileNameOpts=Use function name
      mask Help: web(which(['common_lib44.html']))
      mask TypeOptions DType: double | single
      mask Display:
      | patch([0.3 0.3 0.7 0.7], [0.35 0.65 0.65 0.35], [255/255 127/255 255/255])
      | 
      | plot([.2 .9],[0.5 0.5],[0.2 0.3 0.8 .9],[.25 .25 .75 .75])
      | 
      | port_label('input', 1, 'Y_1')
      | port_label('input', 2, 'Y_0')
      | port_label('input', 3, 'X_1')
      | port_label('input', 4, 'X_0')
      | port_label('input', 5, 'X')

== system common_lib/Timers ==
  note: Timers
  Timer : Subsystem  mask{TimeStep=0}
      mask prompts: TimeStep "Time Step (double)"
      mask help:
      | This block outputs a boolean true when In has been true
      | for at least the TiggerTime time.
